simulink model "DC_Charging_Sequence_Block_complete"  (R2025b)
settings: Solver=FixedStepDiscrete  StartTime=0.0  StopTime=10.0  FixedStep=0.01  RelTol=1e-3
undefined symbols (not defined in the file or in its folder): CCM, raptor_get_safe_string, raptor_xcp_function
libraries: Raptor_lib x32
(part 1 of 2)
settings Model: RaptorUIDSize=4  Raptor_Target=CCM-58NN-112-2403  Raptor_Calloc=NonVolatile (EEPROM)  Raptor_ecuaddr=11  RaptorBuildNum=-1  Creator=noahm  LastModifiedBy=nmonson
settings OptimizationCC: DefaultParameterBehavior=Inlined  UseSpecifiedMinMax=on  InlineInvariantSignals=on  EnhancedBackFolding=on  PassReuseOutputArgsAs=Individual arguments  InitFltsAndDblsToZero=on  NoFixptDivByZeroProtection=on  EfficientFloat2IntCast=on  OptimizeBlockOrder=speed  DifferentSizesBufferReuse=on  OptimizationCustomize=off  EfficientTunableParamExpr=on
settings DebuggingCC: UnderspecifiedInitializationDetection=Classic  MergeDetectMultiDrivingBlocksExec=none  InheritedTsInSrcMsg=none  ParameterTunabilityLossMsg=error
settings HardwareCC: TargetIntDivRoundTo=Zero  TargetEndianess=BigEndian  ProdEqTarget=off
settings ModelReferenceCC: PropagateSignalLabelsOutOfModel=off
settings SFSimCC: MATLABDynamicMemAlloc=off
settings RTWCC: SystemTargetFile=raptor.tlc  MakeCommand=raptor_make_rtw  TemplateMakefile=raptor_tmf  Description=Raptor (tm)
settings CodeAppCC: ForceParamTrailComments=on  IgnoreCustomStorageClasses=off  MaxIdLength=100.0  OperatorAnnotations=on  SimulinkDataObjDesc=on  SFDataObjDesc=on  InsertBlockDesc=on
settings STFCustomTargetCC: SystemTargetFile=raptor.tlc  TargetLangStandard=C99 (ISO)  MultiwordLength=256.0  GenerateSampleERTMain=on  ConcurrentExecutionCompliant=off  CombineOutputUpdateFcns=on  CombineSignalStateStructs=on  ERTCustomFileBanners=on  SupportComplex=off  SupportContinuousTime=off  SupportNonInlinedSFcns=off  RemoveResetFunc=on  MATLABClassNameForMDSCustomization=Simulink.SoftwareTarget.ERTCustomization  GRTInterface=off  raptor_autosave=on  raptor_pack_rtw=off
settings ERTTargetCC: ERTCustomFileTemplate=example_file_process.tlc  TargetLangStandard=C99 (ISO)  GenerateSampleERTMain=on  ParMdlRefBuildCompliant=off  CompOptLevelCompliant=off  ConcurrentExecutionCompliant=off  CombineSignalStateStructs=on  SupportComplex=off  ModelStepFunctionPrototypeControlCompliant=off  CPPClassGenCompliant=off  UseToolchainInfoCompliant=off

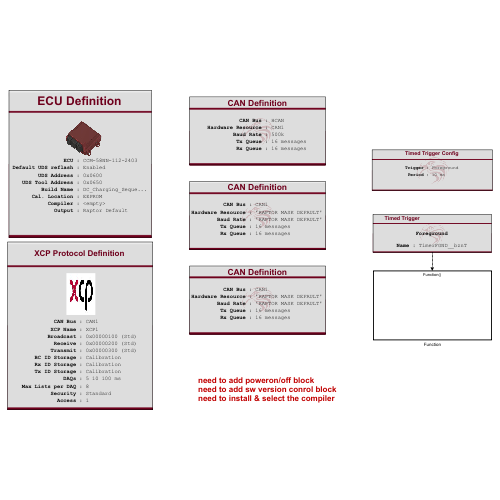
[thumbnail: Simulink's stored preview of the top-level diagram]
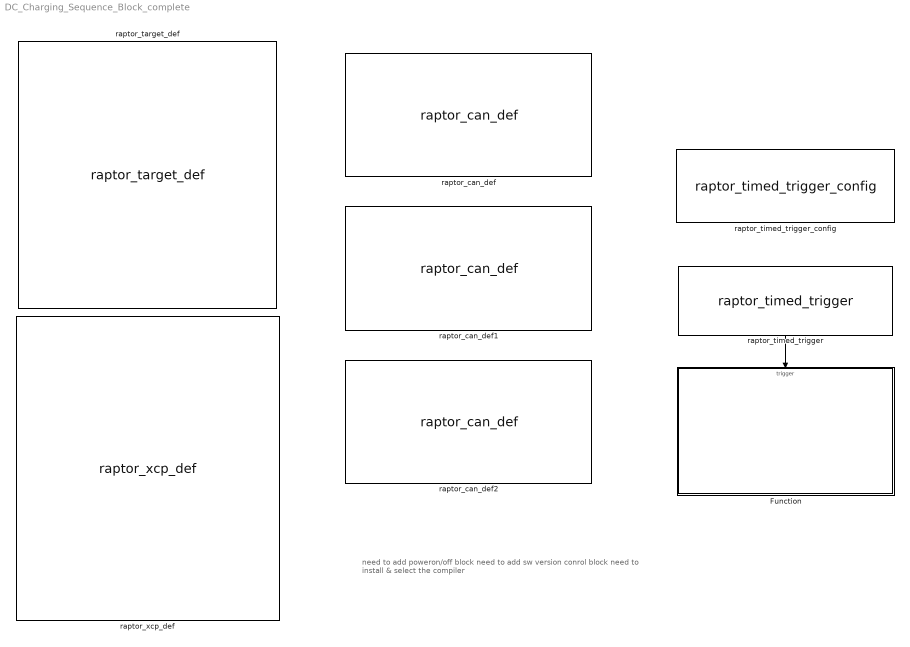
== system DC_Charging_Sequence_Block_complete ==
  note: need to add poweron/off block
      | need to add sw version conrol block
      | need to install & select the compiler
  Function : Subsystem
  raptor_can_def : Raptor_lib/CAN/raptor_can_def  canBus='HCAN'  resourceValues=CAN1|CAN2|CAN3|CAN4|CAN5|CAN6|CAN7|CAN8|(None)  resource=CAN1  baudRateValues=33k|50k|100k|125k|200k|250k|333k|500k|667k|800k|1000k  baudRate=500k  useCustomBR=0  customBR='CustomBaudRate'  enable_baud_rate_config=0  sim_func_name='ConfigureCANBaudRate'  createButton=0  updateButton=0  txQueueSize=16  rxQueueSize=16
      settings: SourceProductName=Raptor
  raptor_can_def1 : Raptor_lib/CAN/raptor_can_def  canBus='CAN1'  resourceValues=CAN1|CAN2|CAN3|CAN4|CAN5|CAN6|CAN7|CAN8|(None)  resource='RAPTOR MASK DEFAULT'  baudRateValues=(None)  baudRate='RAPTOR MASK DEFAULT'  useCustomBR=0  customBR='CustomBaudRate'  enable_baud_rate_config=0  sim_func_name='ConfigureCANBaudRate'  createButton=[]  updateButton=[]  txQueueSize=16  rxQueueSize=16
      settings: SourceProductName=Raptor
  raptor_can_def2 : Raptor_lib/CAN/raptor_can_def  canBus='CAN1'  resourceValues=CAN1|CAN2|CAN3|CAN4|CAN5|CAN6|CAN7|CAN8|(None)  resource='RAPTOR MASK DEFAULT'  baudRateValues=(None)  baudRate='RAPTOR MASK DEFAULT'  useCustomBR=0  customBR='CustomBaudRate'  enable_baud_rate_config=0  sim_func_name='ConfigureCANBaudRate'  createButton=[]  updateButton=[]  txQueueSize=16  rxQueueSize=16
      settings: SourceProductName=Raptor
  raptor_target_def : Raptor_lib/Configuration/raptor_target_def  targetValues=CCM-58NN-112-2403|CCM-TC377-112-2403|DISP-VC128-1901|DISP-VC320L-1402|DISP-VC320-1204|DISP-VC800-1402|DISP-VC500-1904|DISP-VC700-2003|DISP-VC300R-2004|GCM-5634M-070-1559|GCM-5634M-070-1562|EOL-58NN-176-2204|ECM-1793-196-1503|GCM-1793-196-1503|GCM-5605B-048-1906|GCM-5605B-048-2104|RCM-5743R-080-2203|RCM-5743R-080-2304|UAS-5743R-047-2102|UAS-5743R-047-2107|RCM-58NN-112-2103|RCM-58NN-112-2202|RCM-58NN-112-2208|RCM-58NN-112-2410|GCM-TC234-044-2409|GCM-TC277-106-2407|GCM-TC277-108-2406|GCM-TC337-056-2402|GCM-TC367-111-2301|HCM-5604-036-1303|HCM-5604-036-1702  target=CCM-58NN-112-2403  simpack=0  simulator=0  heap=2*1024  stack=4*1024  fgndStack=2*1024  bgndStack=2*1024  idleStack=1024  intStack=1536  sdStack=1024  appStack=1024  ecuaddr=11  disable_def_uds_reflash=0  uds_server_addr_ext=0  uds_server_addr=hex2dec('600')  uds_client_addr=hex2dec('650')  callocValues=Constant (FLASH)|NonVolatile (EEPROM)  calloc=NonVolatile (EEPROM)  compilerValues=[]  compiler=<empty>  setFileName=0  exeName=[raptor_get_safe_string(bdroot) '_']  addBuildNum=0  minVerChars=3  extraOutput=1  buildLocationValues=Raptor Default|Model Directory|User Defined  buildLocation=Raptor Default  exeLocation=''  exeFileButton=0  a2lLocation=''  a2lFileButton=0  rpgLocation=''  rpgFileButton=0
      settings: SourceProductName=Raptor
  raptor_timed_trigger : Raptor_lib/Triggers/raptor_timed_trigger  triggerValues=[]  trigger=Foreground  inherited=0  alwaysEnabled=1  triggerPriority=0  triggerName=FGND__bznT
      settings: SourceProductName=Raptor
  raptor_timed_trigger_config : Raptor_lib/Triggers/raptor_timed_trigger_config  triggerValues=Foreground|Background  trigger=Foreground  period=10
      settings: SourceProductName=Raptor
  raptor_xcp_def : Raptor_lib/Configuration/raptor_xcp_def  XCPname='XCP1'  canBus='CAN1'  bcID=hex2dec('100')  bcID_TypeValues=[]  bcID_Type=Standard  rxID=hex2dec('200')  rxID_TypeValues=[]  rxID_Type=Standard  txID=hex2dec('300')  txID_TypeValues=[]  txID_Type=Standard  daqRates=[5 10 100]  numODTs=8  genCANAPE=0  genVISION=0  securityValues=[]  security=Standard  dllName=raptor_XCPSecurity.dll  accessValues=[]  access=1  bcStorageValues=[]  bcStorage=Calibration  txStorageValues=[]  txStorage=Calibration  rxStorageValues=[]  rxStorage=Calibration
      settings: SourceProductName=Raptor
  wires:
  raptor_timed_trigger/1 -> Function/Trigger

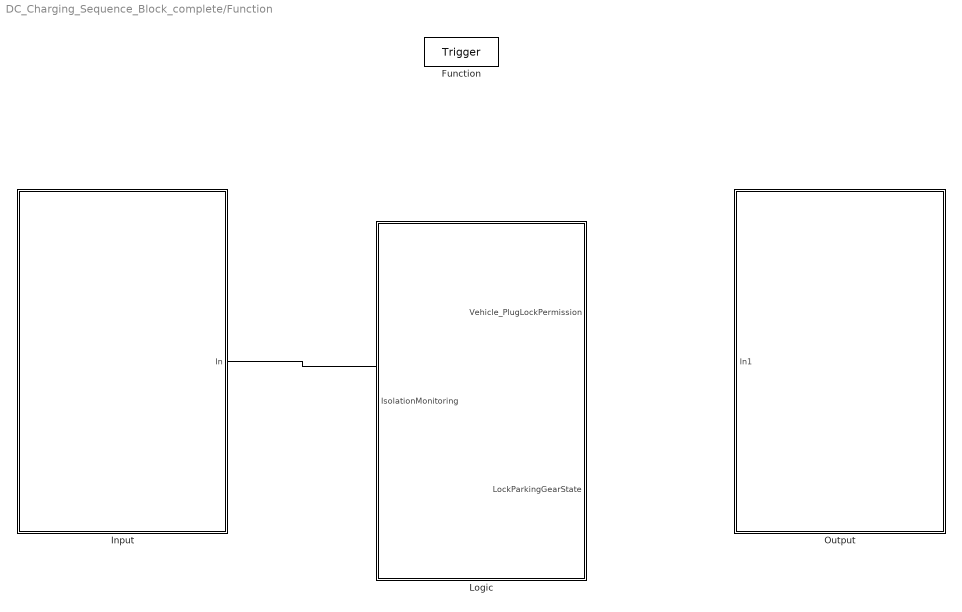
== system DC_Charging_Sequence_Block_complete/Function ==
  Function : TriggerPort  TriggerType=function-call  VariantControl=(inherit)  PortDimensions=1
  Input : Subsystem
  Logic : Subsystem
  Output : Subsystem
  wires:
  Input/1(In) -> ?
  ? -> Output/1(In1)

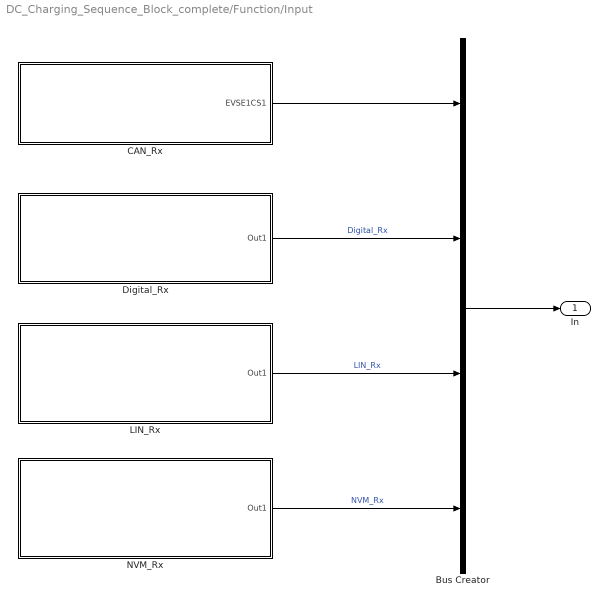
== system DC_Charging_Sequence_Block_complete/Function/Input ==
  Bus Creator : BusCreator  Inputs=4
  CAN_Rx : Subsystem
  Digital_Rx : Subsystem
  LIN_Rx : Subsystem
  NVM_Rx : Subsystem
  In : Outport
  wires:
  Digital_Rx/1(Out1) -> Bus Creator/2  "Digital_Rx"
  LIN_Rx/1(Out1) -> Bus Creator/3  "LIN_Rx"
  NVM_Rx/1(Out1) -> Bus Creator/4  "NVM_Rx"
  Bus Creator/1 -> In/1
  CAN_Rx/1(EVSE1CS1) -> Bus Creator/1

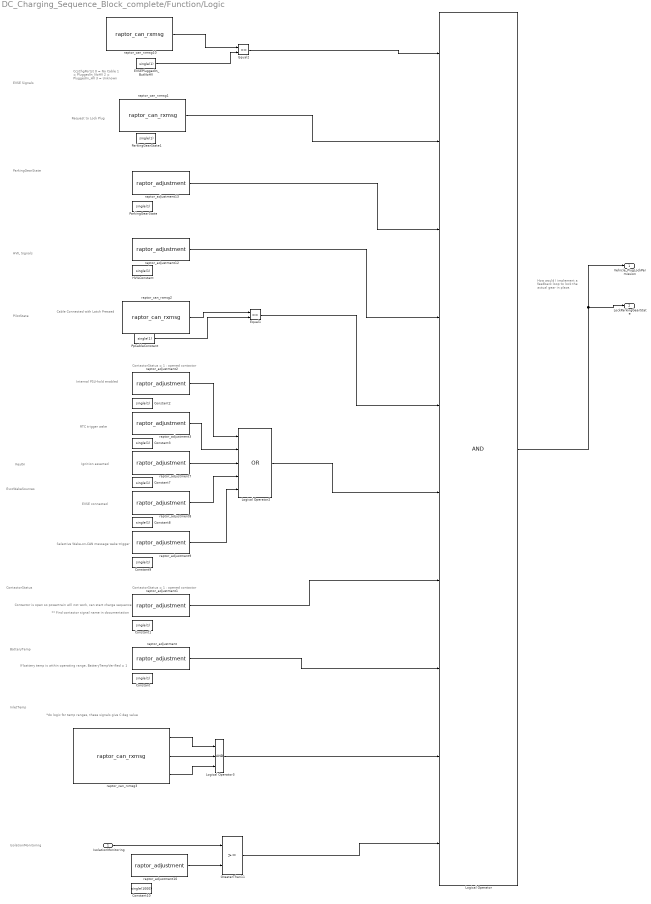
== system DC_Charging_Sequence_Block_complete/Function/Logic ==
  note: Selective Wake-on-CAN message wake trigger
  note: EVSE connected
  note: Ignition asserted
  note: RTC trigger wake
  note: Internal PSU-hold enabled
  note: *do logic for temp ranges, these signals give C deg value
  note: If battery temp is within operating range, BatteryTempVerified = 1
  note: ContactorStatus
  note: EVSE Signals
  note: ParkingGearState
  note: How would I implement a feedback loop to lock the actual gear in place.
  note: Request to Lock Plug
  note: HVIL Signals
  note: PilotState
  note: KeyOn
  note: EvccWakeSources
  note: Contactor is open so powertrain will not work, can start charge sequence
  note: ContactorStatus = 1 : opened contactor
  note: ** Find contactor signal name in documentation
  note: BatteryTemp
  note: InletTemp
  note: IsolationMonitoring
  note: ContactorStatus = 1 : opened contactor
  note: Cable Connected with Latch Pressed
  note: CcsChgPortst
      | 0 = No Cable
      | 1 = PluggedIn_NoHV
      | 2 = PluggedIn_HV
      | 3 = Unknown
  IsolationMonitoring : Inport
  Constant{,1..3,7..9} (7 alike) : Constant  Value=single(1)
  Constant10 : Constant  Value=single(1000)
  EVSEPluggedIn_ButNoHV : Constant  Value=single(1)
  Equal1 : RelationalOperator  Operator===  OutDataTypeStr=boolean  RndMeth=Simplest  InputSameDT=off
  Equal2 : RelationalOperator  Operator===  OutDataTypeStr=boolean  RndMeth=Simplest  InputSameDT=off
  GreaterThan11 : RelationalOperator  OutDataTypeStr=boolean  RndMeth=Simplest  InputSameDT=off
  HVILConstant : Constant  Value=single(1)
  Logical Operator : Logic  Inputs=10  AllPortsSameDT=off  OutDataTypeStr=boolean
  Logical Operator2 : Logic  Operator=OR  Inputs=5  AllPortsSameDT=off  OutDataTypeStr=boolean
  Logical Operator3 : Logic  Inputs=3  AllPortsSameDT=off  OutDataTypeStr=boolean
  ParkingGearState : Constant  Value=single(1)
  ParkingGearState1 : Constant  Value=single(1)
  PpCableConstant : Constant  Value=single(1)
  raptor_adjustment : Raptor_lib/Data Storage/raptor_adjustment  paramName='BatteryTempVerified'  nameSource=Parameter  initValue=1  dataType=single  storage=Calibration  calDispType=Number  calEnum={'False', 'True'}  calGain=1.0  calOffset=0.0  calMax=inf  calMin=-inf  calFormat='-1'  calUnit=''  calHelp=''  calAccess=1  calFunction=raptor_xcp_function(gcb)  calDispHeaders=off  calColHeaders={'Col1' 'Col2' 'Col3'}  calRowHeaders={'Row1' 'Row2' 'Row3'}
      settings: SourceProductName=Raptor
  raptor_adjustment1 : Raptor_lib/Data Storage/raptor_adjustment  paramName='ContactorStatus1'  nameSource=Parameter  initValue=1  dataType=single  storage=Calibration  calDispType=Number  calEnum={'False', 'True'}  calGain=1.0  calOffset=0.0  calMax=inf  calMin=-inf  calFormat='-1'  calUnit=''  calHelp=''  calAccess=1  calFunction=raptor_xcp_function(gcb)  calDispHeaders=off  calColHeaders={'Col1' 'Col2' 'Col3'}  calRowHeaders={'Row1' 'Row2' 'Row3'}
      settings: SourceProductName=Raptor
  raptor_adjustment10 : Raptor_lib/Data Storage/raptor_adjustment  paramName='IsolationMonitoringConstant'  nameSource=Parameter  initValue=1000  dataType=single  storage=Calibration  calDispType=Number  calEnum={'False', 'True'}  calGain=1.0  calOffset=0.0  calMax=inf  calMin=-inf  calFormat='-1'  calUnit=''  calHelp=''  calAccess=1  calFunction=raptor_xcp_function(gcb)  calDispHeaders=off  calColHeaders={'Col1' 'Col2' 'Col3'}  calRowHeaders={'Row1' 'Row2' 'Row3'}
      settings: SourceProductName=Raptor
  raptor_adjustment12 : Raptor_lib/Data Storage/raptor_adjustment  paramName='HVIL_sim'  nameSource=Parameter  initValue=1  dataType=single  storage=Calibration  calDispType=Enumeration  calEnum={'Cable Disconnected', 'Cable Connected with Latch Pressed', 'Cable Connected with Latch Released', 'Proximity Signal is invalid'}  calGain=1.0  calOffset=0.0  calMax=inf  calMin=-inf  calFormat='-1'  calUnit=''  calHelp=''  calAccess=1  calFunction=raptor_xcp_function(gcb)  calDispHeaders=off  calColHeaders={'Col1' 'Col2' 'Col3'}  calRowHeaders={'Row1' 'Row2' 'Row3'}
      settings: SourceProductName=Raptor
  raptor_adjustment13 : Raptor_lib/Data Storage/raptor_adjustment  paramName='ParkingGear_sim'  nameSource=Parameter  initValue=1  dataType=single  storage=Calibration  calDispType=Enumeration  calEnum={'Cable Disconnected', 'Cable Connected with Latch Pressed', 'Cable Connected with Latch Released', 'Proximity Signal is invalid'}  calGain=1.0  calOffset=0.0  calMax=inf  calMin=-inf  calFormat='-1'  calUnit=''  calHelp=''  calAccess=1  calFunction=raptor_xcp_function(gcb)  calDispHeaders=off  calColHeaders={'Col1' 'Col2' 'Col3'}  calRowHeaders={'Row1' 'Row2' 'Row3'}
      settings: SourceProductName=Raptor
  raptor_adjustment2 : Raptor_lib/Data Storage/raptor_adjustment  paramName='EvccWakeSources1_sim'  nameSource=Parameter  initValue=1  dataType=single  storage=Calibration  calDispType=Number  calEnum={'False', 'True'}  calGain=1.0  calOffset=0.0  calMax=inf  calMin=-inf  calFormat='-1'  calUnit=''  calHelp=''  calAccess=1  calFunction=raptor_xcp_function(gcb)  calDispHeaders=off  calColHeaders={'Col1' 'Col2' 'Col3'}  calRowHeaders={'Row1' 'Row2' 'Row3'}
      settings: SourceProductName=Raptor
  raptor_adjustment3 : Raptor_lib/Data Storage/raptor_adjustment  paramName='EvccWakeSources2_sim'  nameSource=Parameter  initValue=1  dataType=single  storage=Calibration  calDispType=Number  calEnum={'False', 'True'}  calGain=1.0  calOffset=0.0  calMax=inf  calMin=-inf  calFormat='-1'  calUnit=''  calHelp=''  calAccess=1  calFunction=raptor_xcp_function(gcb)  calDispHeaders=off  calColHeaders={'Col1' 'Col2' 'Col3'}  calRowHeaders={'Row1' 'Row2' 'Row3'}
      settings: SourceProductName=Raptor
  raptor_adjustment7 : Raptor_lib/Data Storage/raptor_adjustment  paramName='EvccWakeSources3_sim'  nameSource=Parameter  initValue=1  dataType=single  storage=Calibration  calDispType=Number  calEnum={'False', 'True'}  calGain=1.0  calOffset=0.0  calMax=inf  calMin=-inf  calFormat='-1'  calUnit=''  calHelp=''  calAccess=1  calFunction=raptor_xcp_function(gcb)  calDispHeaders=off  calColHeaders={'Col1' 'Col2' 'Col3'}  calRowHeaders={'Row1' 'Row2' 'Row3'}
      settings: SourceProductName=Raptor
  raptor_adjustment8 : Raptor_lib/Data Storage/raptor_adjustment  paramName='EvccWakeSources4_sim'  nameSource=Parameter  initValue=1  dataType=single  storage=Calibration  calDispType=Number  calEnum={'False', 'True'}  calGain=1.0  calOffset=0.0  calMax=inf  calMin=-inf  calFormat='-1'  calUnit=''  calHelp=''  calAccess=1  calFunction=raptor_xcp_function(gcb)  calDispHeaders=off  calColHeaders={'Col1' 'Col2' 'Col3'}  calRowHeaders={'Row1' 'Row2' 'Row3'}
      settings: SourceProductName=Raptor
  raptor_adjustment9 : Raptor_lib/Data Storage/raptor_adjustment  paramName='EvccWakeSources5_sim'  nameSource=Parameter  initValue=1  dataType=single  storage=Calibration  calDispType=Number  calEnum={'False', 'True'}  calGain=1.0  calOffset=0.0  calMax=inf  calMin=-inf  calFormat='-1'  calUnit=''  calHelp=''  calAccess=1  calFunction=raptor_xcp_function(gcb)  calDispHeaders=off  calColHeaders={'Col1' 'Col2' 'Col3'}  calRowHeaders={'Row1' 'Row2' 'Row3'}
      settings: SourceProductName=Raptor
  raptor_can_rxmsg1 : Raptor_lib/CAN/raptor_can_rxmsg  canDefinition=struct('dbcFile', 'CCU_VehicleInterface_R5371_matlab.dbc','message', 'EVCC_Sequence','comment', '','signals', {{'CcsChgPortLockStReq','CcsChgRlyStReq','CcsEvIsolStopReq','CcsRlyWeldCheckEn','Checksum','Counter'}},'enabled', [ 1 0 0 0 0 0;],'scaled', [ 1 1 1 1 1 1;],'canBus', '''CAN1''','messageID', [ 419414367;],'idMask', [ 536870911;],'payloadMask', [],'payloadValue', [],'period', [ 0;],'mailbox', '''''','queueSize', [ 1;],'label', [ 1;],'ver', [ 2;],'showID', [ 0;],'showRaw', [ 0;],'showRawMsg', [ 0;],'useStartVals', [ 0;],'extendedId', [ 1;],'showAge', [ 0;],'useSimFunc', [ 0;],'sim_func_name', '''''','fill', [ 0;],'editID', [ 0;],'signalOrder', [ 1;],'signalAscDes', [ 1;],'msgLength', [ 3;])  canBus='CAN1'  mailbox=''  payloadMask=[]  payloadValue=[]  idMask=hex2dec('1FFFFFFF')  queueSize=1  showID=0  label=1  fill=0  id=419414367  showRaw=0  showAge=0  signalOrder=1  signalInfo={{struct('Name', 'CcsChgPortLockStReq','StartBit', [ 2;],'SignalSize', [ 2;],'ByteOrder', 'LittleEndian','ValueType', 'Integer','Class', 'uint8','Signed', '0','Factor', [ 1;],'Offset', [ 0;],'Min', [ 0;],'Max', [ 3;],'Units', 'bool','Comment', 'Desired status of charge port lock. TRUE value is a request to lock the port and FALSE value is a request to unlock it','Multiplexor', [ 0;],'Multiplexed', [ 0;],'Muxor_Name', '','MultiplexMode_Min', [],'MultiplexMode_Max', [],'StartVal', [ 0;]),struct('Name', 'CcsChgRlyStReq','StartBit', [ 4;],'SignalSize', [ 2;],'ByteOrder', 'LittleEndian','ValueType', 'Integer','Class', 'uint8','Signed', '0','Factor', [ 1;],'Offset', [ 0;],'Min', [ 0;],'Max', [ 3;],'Units', 'bool','Comment', 'Desired relay status request from PI-EVCC; TRUE value is a request to close the relay;','Multiplexor', [ 0;],'Multiplexed', [ 0;],'Muxor_Name', '','MultiplexMode_Min', [],'MultiplexMode_Max', [],'StartVal', [ 0;]),struct('Name', 'CcsEvIsolStopReq','StartBit', [ 0;],'SignalSize', [ 2;],'ByteOrder', 'LittleEndian','ValueType', 'Integer','Class', 'uint8','Signed', '0','Factor', [ 1;],'Offset', [ 0;],'Min', [ 0;],'Max', [ 3;],'Units', 'bool','Comment', 'TRUE value is a Request from PI-EVCC for EV to stop HV Isolation monitoring','Multiplexor', [ 0;],'Multiplexed', [ 0;],'Muxor_Name', '','MultiplexMode_Min', [],'MultiplexMode_Max', [],'StartVal', [ 0;]),struct('Name', 'CcsRlyWeldCheckEn','StartBit', [ 6;],'SignalSize', [ 2;],'ByteOrder', 'LittleEndian','ValueType', 'Integer','Class', 'uint8','Signed', '0','Factor', [ 1;],'Offset', [ 0;],'Min', [ 0;],'Max', [ 3;],'Units', 'bool','Comment', 'Charging session sequence of events: TRUE value is to notify EV that the logic for relay weld-checking can be executed','Multiplexor', [ 0;],'Multiplexed', [ 0;],'Muxor_Name', '','MultiplexMode_Min', [],'MultiplexMode_Max', [],'StartVal', [ 0;]),struct('Name', 'Checksum','StartBit', [ 16;],'SignalSize', [ 8;],'ByteOrder', 'LittleEndian','ValueType', 'Integer','Class', 'uint8','Signed', '0','Factor', [ 1;],'Offset', [ 0;],'Min', [ 0;],'Max', [ 255;],'Units', 'NU','Comment', 'CAN message checksum','Multiplexor', [ 0;],'Multiplexed', [ 0;],'Muxor_Name', '','MultiplexMode_Min', [],'MultiplexMode_Max', [],'StartVal', [ 0;]),struct('Name', 'Counter','StartBit', [ 12;],'SignalSize', [ 4;],'ByteOrder', 'LittleEndian','ValueType', 'Integer','Class', 'uint8','Signed', '0','Factor', [ 1;],'Offset', [ 0;],'Min', [ 0;],'Max', [ 0;],'Units', '','Comment', 'CAN message sequence counter','Multiplexor', [ 0;],'Multiplexed', [ 0;],'Muxor_Name', '','MultiplexMode_Min', [],'MultiplexMode_Max', [],'StartVal', [ 0;])}}  showRawMsg=0  useSimFunc=0  sim_func_name=''  useStartVals=0  extendedId=1
      settings: SourceProductName=Raptor
  raptor_can_rxmsg10 : Raptor_lib/CAN/raptor_can_rxmsg  canDefinition=struct('dbcFile', 'CCU_VehicleInterface_R5371_matlab.dbc','message', 'EVCC_Status','comment', '','signals', {{'CcsChargingMode','CcsChgPortSt','CcsChgSessionPhase','CcsCpState','CcsSelectedControlMode','CcsSelectedProtocol','CcsSelectedServiceId','Checksum','Counter','FaultCode','FaultWord'}},'enabled', [ 0 1 0 0 0 0 0 0 0 0 0;],'scaled', [ 1 1 1 1 1 1 1 1 1 1 1;],'canBus', '''CAN1''','messageID', [ 419414111;],'idMask', [ 536870911;],'payloadMask', [],'payloadValue', [],'period', [ 0;],'mailbox', '''''','queueSize', [ 1;],'label', [ 1;],'ver', [ 2;],'showID', [ 0;],'showRaw', [ 0;],'showRawMsg', [ 0;],'useStartVals', [ 0;],'extendedId', [ 1;],'showAge', [ 0;],'useSimFunc', [ 0;],'sim_func_name', '''''','fill', [ 0;],'editID', [ 0;],'signalOrder', [ 1;],'signalAscDes', [ 1;],'msgLength', [ 8;])  canBus='CAN1'  mailbox=''  payloadMask=[]  payloadValue=[]  idMask=hex2dec('1FFFFFFF')  queueSize=1  showID=0  label=1  fill=0  id=419414111  showRaw=0  showAge=0  signalOrder=1  signalInfo={{struct('Name', 'CcsChargingMode','StartBit', [ 12;],'SignalSize', [ 4;],'ByteOrder', 'LittleEndian','ValueType', 'Integer','Class', 'uint8','Signed', '0','Factor', [ 1;],'Offset', [ 0;],'Min', [ 0;],'Max', [ 15;],'Units', '','Comment', 'Charging mode identified by EVCC based on Control Pilot (CP) PWM input','Multiplexor', [ 0;],'Multiplexed', [ 0;],'Muxor_Name', '','MultiplexMode_Min', [],'MultiplexMode_Max', [],'StartVal', [ 0;]),struct('Name', 'CcsChgPortSt','StartBit', [ 0;],'SignalSize', [ 2;],'ByteOrder', 'LittleEndian','ValueType', 'Integer','Class', 'uint8','Signed', '0','Factor', [ 1;],'Offset', [ 0;],'Min', [ 0;],'Max', [ 3;],'Units', 'enum','Comment', 'The status of charging port (plugged, unplugged, unknown).','Multiplexor', [ 0;],'Multiplexed', [ 0;],'Muxor_Name', '','MultiplexMode_Min', [],'MultiplexMode_Max', [],'StartVal', [ 0;]),struct('Name', 'CcsChgSessionPhase','StartBit', [ 2;],'SignalSize', [ 6;],'ByteOrder', 'LittleEndian','ValueType', 'Integer','Class', 'uint8','Signed', '0','Factor', [ 1;],'Offset', [ 0;],'Min', [ 0;],'Max', [ 63;],'Units', 'No Unit','Comment', 'a number that indicates the current phase of charging session as well as charging mode (AC or DC). See user guide document to interpret the number','Multiplexor', [ 0;],'Multiplexed', [ 0;],'Muxor_Name', '','MultiplexMode_Min', [],'MultiplexMode_Max', [],'StartVal', [ 0;]),struct('Name', 'CcsCpState','StartBit', [ 8;],'SignalSize', [ 4;],'ByteOrder', 'LittleEndian','ValueType', 'Integer','Class', 'uint8','Signed', '0','Factor', [ 1;],'Offset', [ 0;],'Min', [ 0;],'Max', [ 15;],'Units', '','Comment', 'State of Control Pilot (CP) signal','Multiplexor', [ 0;],'Multiplexed', [ 0;],'Muxor_Name', '','MultiplexMode_Min', [],'MultiplexMode_Max', [],'StartVal', [ 0;]),struct('Name', 'CcsSelectedControlMode','StartBit', [ 51;],'SignalSize', [ 1;],'ByteOrder', 'LittleEndian','ValueType', 'Integer','Class', 'uint8','Signed', '0','Factor', [ 1;],'Offset', [ 0;],'Min', [ 0;],'Max', [ 1;],'Units', '','Comment', 'Control Mode selected during ISO15118-20 HLC session; 1 = Dynamic control mode, 0 = Schedule control mode','Multiplexor', [ 0;],'Multiplexed', [ 0;],'Muxor_Name', '','MultiplexMode_Min', [],'MultiplexMode_Max', [],'StartVal', [ 0;]),struct('Name', 'CcsSelectedProtocol','StartBit', [ 40;],'SignalSize', [ 3;],'ByteOrder', 'LittleEndian','ValueType', 'Integer','Class', 'uint8','Signed', '0','Factor', [ 1;],'Offset', [ 0;],'Min', [ 0;],'Max', [ 7;],'Units', '','Comment', 'Protocol selected after exchanging SupportedAppProtocolReq/Res pair','Multiplexor', [ 0;],'Multiplexed', [ 0;],'Muxor_Name', '','MultiplexMode_Min', [],'MultiplexMode_Max', [],'StartVal', [ 0;]),struct('Name', 'CcsSelectedServiceId','StartBit', [ 43;],'SignalSize', [ 8;],'ByteOrder', 'LittleEndian','ValueType', 'Integer','Class', 'uint8','Signed', '0','Factor', [ 1;],'Offset', [ 0;],'Min', [ 0;],'Max', [ 255;],'Units', '','Comment', 'Service ID selected during an HLC session; DC_Charging (2), DC_BPT (17)','Multiplexor', [ 0;],'Multiplexed', [ 0;],'Muxor_Name', '','MultiplexMode_Min', [],'MultiplexMode_Max', [],'StartVal', [ 0;]),struct('Name', 'Checksum','StartBit', [ 56;],'SignalSize', [ 8;],'ByteOrder', 'LittleEndian','ValueType', 'Integer','Class', 'uint8','Signed', '0','Factor', [ 1;],'Offset', [ 0;],'Min', [ 0;],'Max', [ 255;],'Units', 'NU','Comment', 'CAN message checksum','Multiplexor', [ 0;],'Multiplexed', [ 0;],'Muxor_Name', '','MultiplexMode_Min', [],'MultiplexMode_Max', [],'StartVal', [ 0;]),struct('Name', 'Counter','StartBit', [ 52;],'SignalSize', [ 4;],'ByteOrder', 'LittleEndian','ValueType', 'Integer','Class', 'uint8','Signed', '0','Factor', [ 1;],'Offset', [ 0;],'Min', [ 0;],'Max', [ 0;],'Units', '','Comment', 'CAN message sequence counter','Multiplexor', [ 0;],'Multiplexed', [ 0;],'Muxor_Name', '','MultiplexMode_Min', [],'MultiplexMode_Max', [],'StartVal', [ 0;]),struct('Name', 'FaultCode','StartBit', [ 16;],'SignalSize', [ 16;],'ByteOrder', 'LittleEndian','ValueType', 'Integer','Class', 'uint16','Signed', '0','Factor', [ 1;],'Offset', [ 0;],'Min', [ 0;],'Max', [ 65535;],'Units', 'NU','Comment', 'A code that indicates the presence of an active fault related to communication with EV or PiEVCC pins or any fault that is not directly related to EVSE interface','Multiplexor', [ 0;],'Multiplexed', [ 0;],'Muxor_Name', '','MultiplexMode_Min', [],'MultiplexMode_Max', [],'StartVal', [ 0;]),struct('Name', 'FaultWord','StartBit', [ 32;],'SignalSize', [ 8;],'ByteOrder', 'LittleEndian','ValueType', 'Integer','Class', 'uint8','Signed', '0','Factor', [ 1;],'Offset', [ 0;],'Min', [ 0;],'Max', [ 255;],'Units', 'NU','Comment', 'Fault word with each bit representing a particular type of fault','Multiplexor', [ 0;],'Multiplexed', [ 0;],'Muxor_Name', '','MultiplexMode_Min', [],'MultiplexMode_Max', [],'StartVal', [ 0;])}}  showRawMsg=0  useSimFunc=0  sim_func_name=''  useStartVals=0  extendedId=1
      settings: SourceProductName=Raptor
  raptor_can_rxmsg2 : Raptor_lib/CAN/raptor_can_rxmsg  canDefinition=struct('dbcFile', 'CCU_VehicleInterface_R5371_matlab.dbc','message', 'EVCC_IOandWake_Info','comment', '','signals', {{'CcsPpState','Checksum','Counter','Din2St','DoutHsd1St','DoutHsd2St','DoutLsd1St','DoutLsd2St','DoutLsd3St','DoutLsd4St','DoutLsd5St','EvccWakeSources','Hbrg1_Curr','InletLockSt','Rly1FdbkSt','Rly2FdbkSt'}},'enabled', [ 1 0 0 0 0 0 0 0 0 0 0 0 0 0 0 0;],'scaled', [ 1 1 1 1 1 1 1 1 1 1 1 1 1 1 1 1;],'canBus', '''CAN1''','messageID', [ 419416671;],'idMask', [ 536870911;],'payloadMask', [],'payloadValue', [],'period', [ 0;],'mailbox', '''''','queueSize', [ 1;],'label', [ 1;],'ver', [ 2;],'showID', [ 0;],'showRaw', [ 0;],'showRawMsg', [ 0;],'useStartVals', [ 0;],'extendedId', [ 1;],'showAge', [ 0;],'useSimFunc', [ 0;],'sim_func_name', '''''','fill', [ 0;],'editID', [ 0;],'signalOrder', [ 1;],'signalAscDes', [ 1;],'msgLength', [ 7;])  canBus='CAN1'  mailbox=''  payloadMask=[]  payloadValue=[]  idMask=hex2dec('1FFFFFFF')  queueSize=1  showID=0  label=1  fill=0  id=419416671  showRaw=0  showAge=0  signalOrder=1  signalInfo={{struct('Name', 'CcsPpState','StartBit', [ 39;],'SignalSize', [ 3;],'ByteOrder', 'LittleEndian','ValueType', 'Integer','Class', 'uint8','Signed', '0','Factor', [ 1;],'Offset', [ 0;],'Min', [ 0;],'Max', [ 7;],'Units', '','Comment', 'State of Proximity (PP) signal','Multiplexor', [ 0;],'Multiplexed', [ 0;],'Muxor_Name', '','MultiplexMode_Min', [],'MultiplexMode_Max', [],'StartVal', [ 0;]),struct('Name', 'Checksum','StartBit', [ 48;],'SignalSize', [ 8;],'ByteOrder', 'LittleEndian','ValueType', 'Integer','Class', 'uint8','Signed', '0','Factor', [ 1;],'Offset', [ 0;],'Min', [ 0;],'Max', [ 255;],'Units', 'NU','Comment', 'CAN message checksum','Multiplexor', [ 0;],'Multiplexed', [ 0;],'Muxor_Name', '','MultiplexMode_Min', [],'MultiplexMode_Max', [],'StartVal', [ 0;]),struct('Name', 'Counter','StartBit', [ 44;],'SignalSize', [ 4;],'ByteOrder', 'LittleEndian','ValueType', 'Integer','Class', 'uint8','Signed', '0','Factor', [ 1;],'Offset', [ 0;],'Min', [ 0;],'Max', [ 0;],'Units', '','Comment', 'CAN message sequence counter','Multiplexor', [ 0;],'Multiplexed', [ 0;],'Muxor_Name', '','MultiplexMode_Min', [],'MultiplexMode_Max', [],'StartVal', [ 0;]),struct('Name', 'Din2St','StartBit', [ 30;],'SignalSize', [ 2;],'ByteOrder', 'LittleEndian','ValueType', 'Integer','Class', 'uint8','Signed', '0','Factor', [ 1;],'Offset', [ 0;],'Min', [ 0;],'Max', [ 3;],'Units', 'NU','Comment', 'The present state of digital input 2','Multiplexor', [ 0;],'Multiplexed', [ 0;],'Muxor_Name', '','MultiplexMode_Min', [],'MultiplexMode_Max', [],'StartVal', [ 0;]),struct('Name', 'DoutHsd1St','StartBit', [ 26;],'SignalSize', [ 2;],'ByteOrder', 'LittleEndian','ValueType', 'Integer','Class', 'uint8','Signed', '0','Factor', [ 1;],'Offset', [ 0;],'Min', [ 0;],'Max', [ 3;],'Units', 'NU','Comment', 'The present state of HSD digital output 1','Multiplexor', [ 0;],'Multiplexed', [ 0;],'Muxor_Name', '','MultiplexMode_Min', [],'MultiplexMode_Max', [],'StartVal', [ 0;]),struct('Name', 'DoutHsd2St','StartBit', [ 28;],'SignalSize', [ 2;],'ByteOrder', 'LittleEndian','ValueType', 'Integer','Class', 'uint8','Signed', '0','Factor', [ 1;],'Offset', [ 0;],'Min', [ 0;],'Max', [ 3;],'Units', 'NU','Comment', 'The present state of HSD digital output 2','Multiplexor', [ 0;],'Multiplexed', [ 0;],'Muxor_Name', '','MultiplexMode_Min', [],'MultiplexMode_Max', [],'StartVal', [ 0;]),struct('Name', 'DoutLsd1St','StartBit', [ 16;],'SignalSize', [ 2;],'ByteOrder', 'LittleEndian','ValueType', 'Integer','Class', 'uint8','Signed', '0','Factor', [ 1;],'Offset', [ 0;],'Min', [ 0;],'Max', [ 3;],'Units', 'NU','Comment', 'The present state of LSD digital output 1','Multiplexor', [ 0;],'Multiplexed', [ 0;],'Muxor_Name', '','MultiplexMode_Min', [],'MultiplexMode_Max', [],'StartVal', [ 0;]),struct('Name', 'DoutLsd2St','StartBit', [ 18;],'SignalSize', [ 2;],'ByteOrder', 'LittleEndian','ValueType', 'Integer','Class', 'uint8','Signed', '0','Factor', [ 1;],'Offset', [ 0;],'Min', [ 0;],'Max', [ 3;],'Units', 'NU','Comment', 'The present state of LSD digital output 2','Multiplexor', [ 0;],'Multiplexed', [ 0;],'Muxor_Name', '','MultiplexMode_Min', [],'MultiplexMode_Max', [],'StartVal', [ 0;]),struct('Name', 'DoutLsd3St','StartBit', [ 20;],'SignalSize', [ 2;],'ByteOrder', 'LittleEndian','ValueType', 'Integer','Class', 'uint8','Signed', '0','Factor', [ 1;],'Offset', [ 0;],'Min', [ 0;],'Max', [ 3;],'Units', 'NU','Comment', 'The present state of LSD digital output 3','Multiplexor', [ 0;],'Multiplexed', [ 0;],'Muxor_Name', '','MultiplexMode_Min', [],'MultiplexMode_Max', [],'StartVal', [ 0;]),struct('Name', 'DoutLsd4St','StartBit', [ 22;],'SignalSize', [ 2;],'ByteOrder', 'LittleEndian','ValueType', 'Integer','Class', 'uint8','Signed', '0','Factor', [ 1;],'Offset', [ 0;],'Min', [ 0;],'Max', [ 3;],'Units', 'NU','Comment', 'The present state of LSD digital output 4','Multiplexor', [ 0;],'Multiplexed', [ 0;],'Muxor_Name', '','MultiplexMode_Min', [],'MultiplexMode_Max', [],'StartVal', [ 0;]),struct('Name', 'DoutLsd5St','StartBit', [ 24;],'SignalSize', [ 2;],'ByteOrder', 'LittleEndian','ValueType', 'Integer','Class', 'uint8','Signed', '0','Factor', [ 1;],'Offset', [ 0;],'Min', [ 0;],'Max', [ 3;],'Units', 'NU','Comment', 'The present state of LSD digital output 5','Multiplexor', [ 0;],'Multiplexed', [ 0;],'Muxor_Name', '','MultiplexMode_Min', [],'MultiplexMode_Max', [],'StartVal', [ 0;]),struct('Name', 'EvccWakeSources','StartBit', [ 8;],'SignalSize', [ 8;],'ByteOrder', 'LittleEndian','ValueType', 'Integer','Class', 'uint8','Signed', '0','Factor', [ 1;],'Offset', [ 0;],'Min', [ 0;],'Max', [ 255;],'Units', '','Comment', 'Wake sources currently detected by EVCC (bit position based, multiple active possible)','Multiplexor', [ 0;],'Multiplexed', [ 0;],'Muxor_Name', '','MultiplexMode_Min', [],'MultiplexMode_Max', [],'StartVal', [ 0;]),struct('Name', 'Hbrg1_Curr','StartBit', [ 0;],'SignalSize', [ 8;],'ByteOrder', 'LittleEndian','ValueType', 'Integer','Class', 'uint8','Signed', '0','Factor', [ 0.1;],'Offset', [ 0;],'Min', [ 0;],'Max', [ 21;],'Units', 'A','Comment', 'estimated current of H-Bridge 1','Multiplexor', [ 0;],'Multiplexed', [ 0;],'Muxor_Name', '','MultiplexMode_Min', [],'MultiplexMode_Max', [],'StartVal', [ 0;]),struct('Name', 'InletLockSt','StartBit', [ 36;],'SignalSize', [ 3;],'ByteOrder', 'LittleEndian','ValueType', 'Integer','Class', 'uint8','Signed', '0','Factor', [ 1;],'Offset', [ 0;],'Min', [ 0;],'Max', [ 7;],'Units', '','Comment', 'State of the inlet lock','Multiplexor', [ 0;],'Multiplexed', [ 0;],'Muxor_Name', '','MultiplexMode_Min', [],'MultiplexMode_Max', [],'StartVal', [ 0;]),struct('Name', 'Rly1FdbkSt','StartBit', [ 32;],'SignalSize', [ 2;],'ByteOrder', 'LittleEndian','ValueType', 'Integer','Class', 'uint8','Signed', '0','Factor', [ 1;],'Offset', [ 0;],'Min', [ 0;],'Max', [ 3;],'Units', 'NU','Comment', 'Present state of feedback from charge relay/ contactor 1','Multiplexor', [ 0;],'Multiplexed', [ 0;],'Muxor_Name', '','MultiplexMode_Min', [],'MultiplexMode_Max', [],'StartVal', [ 0;]),struct('Name', 'Rly2FdbkSt','StartBit', [ 34;],'SignalSize', [ 2;],'ByteOrder', 'LittleEndian','ValueType', 'Integer','Class', 'uint8','Signed', '0','Factor', [ 1;],'Offset', [ 0;],'Min', [ 0;],'Max', [ 3;],'Units', 'NU','Comment', 'Present state of feedback from charge relay/ contactor 2','Multiplexor', [ 0;],'Multiplexed', [ 0;],'Muxor_Name', '','MultiplexMode_Min', [],'MultiplexMode_Max', [],'StartVal', [ 0;])}}  showRawMsg=0  useSimFunc=0  sim_func_name=''  useStartVals=0  extendedId=1
      settings: SourceProductName=Raptor
  raptor_can_rxmsg3 : Raptor_lib/CAN/raptor_can_rxmsg  canDefinition=struct('dbcFile', 'CCU_VehicleInterface_R5371_matlab.dbc','message', 'EVCC_TempSensor','comment', '','signals', {{'AIN1_Temperature','AIN2_Temperature','AIN3_Temperature','Checksum','Counter'}},'enabled', [ 1 1 1 0 0;],'scaled', [ 1 1 1 1 1;],'canBus', '''CAN1''','messageID', [ 419415903;],'idMask', [ 536870911;],'payloadMask', [],'payloadValue', [],'period', [ 0;],'mailbox', '''''','queueSize', [ 1;],'label', [ 1;],'ver', [ 2;],'showID', [ 0;],'showRaw', [ 0;],'showRawMsg', [ 0;],'useStartVals', [ 0;],'extendedId', [ 1;],'showAge', [ 0;],'useSimFunc', [ 0;],'sim_func_name', '''''','fill', [ 0;],'editID', [ 0;],'signalOrder', [ 1;],'signalAscDes', [ 1;],'msgLength', [ 8;])  canBus='CAN1'  mailbox=''  payloadMask=[]  payloadValue=[]  idMask=hex2dec('1FFFFFFF')  queueSize=1  showID=0  label=1  fill=0  id=419415903  showRaw=0  showAge=0  signalOrder=1  signalInfo={{struct('Name', 'AIN1_Temperature','StartBit', [ 0;],'SignalSize', [ 12;],'ByteOrder', 'LittleEndian','ValueType', 'Integer','Class', 'uint16','Signed', '0','Factor', [ 1;],'Offset', [ -40;],'Min', [ -40;],'Max', [ 4000;],'Units', 'degC_or_Ohm','Comment', 'Temperature measured using AIN1; Typically AC pin temperature at charge inlet; Value can be in Ohm (PTC) or degC (other types such as PT1000, NTC, etc.)','Multiplexor', [ 0;],'Multiplexed', [ 0;],'Muxor_Name', '','MultiplexMode_Min', [],'MultiplexMode_Max', [],'StartVal', [ 40;]),struct('Name', 'AIN2_Temperature','StartBit', [ 12;],'SignalSize', [ 8;],'ByteOrder', 'LittleEndian','ValueType', 'Integer','Class', 'uint8','Signed', '0','Factor', [ 1;],'Offset', [ -40;],'Min', [ -40;],'Max', [ 210;],'Units', 'degC','Comment', 'Temperature measured using AIN 2; Typically DC positive pin temperature at charge inlet','Multiplexor', [ 0;],'Multiplexed', [ 0;],'Muxor_Name', '','MultiplexMode_Min', [],'MultiplexMode_Max', [],'StartVal', [ 40;]),struct('Name', 'AIN3_Temperature','StartBit', [ 20;],'SignalSize', [ 8;],'ByteOrder', 'LittleEndian','ValueType', 'Integer','Class', 'uint8','Signed', '0','Factor', [ 1;],'Offset', [ -40;],'Min', [ -40;],'Max', [ 210;],'Units', 'degC','Comment', 'Temperature measured using AIN3; Typically DC negative pin temperature at charge inlet','Multiplexor', [ 0;],'Multiplexed', [ 0;],'Muxor_Name', '','MultiplexMode_Min', [],'MultiplexMode_Max', [],'StartVal', [ 40;]),struct('Name', 'Checksum','StartBit', [ 56;],'SignalSize', [ 8;],'ByteOrder', 'LittleEndian','ValueType', 'Integer','Class', 'uint8','Signed', '0','Factor', [ 1;],'Offset', [ 0;],'Min', [ 0;],'Max', [ 255;],'Units', 'NU','Comment', 'CAN message checksum','Multiplexor', [ 0;],'Multiplexed', [ 0;],'Muxor_Name', '','MultiplexMode_Min', [],'MultiplexMode_Max', [],'StartVal', [ 0;]),struct('Name', 'Counter','StartBit', [ 52;],'SignalSize', [ 4;],'ByteOrder', 'LittleEndian','ValueType', 'Integer','Class', 'uint8','Signed', '0','Factor', [ 1;],'Offset', [ 0;],'Min', [ 0;],'Max', [ 0;],'Units', '','Comment', 'CAN message sequence counter','Multiplexor', [ 0;],'Multiplexed', [ 0;],'Muxor_Name', '','MultiplexMode_Min', [],'MultiplexMode_Max', [],'StartVal', [ 0;])}}  showRawMsg=0  useSimFunc=0  sim_func_name=''  useStartVals=0  extendedId=1
      settings: SourceProductName=Raptor
  Vehicle_PlugLockPermission : Outport
  LockParkingGearState : Outport  Port=2
  wires:
  Logical Operator/1 -> Vehicle_PlugLockPermission/1, LockParkingGearState/1
  Equal2/1 -> Logical Operator/1
  Logical Operator2/1 -> Logical Operator/6
  raptor_adjustment10/1 -> GreaterThan11/2
  IsolationMonitoring/1 -> GreaterThan11/1
  GreaterThan11/1 -> Logical Operator/10
  raptor_adjustment1/1 -> Logical Operator/7
  raptor_can_rxmsg3/2 -> Logical Operator3/2
  raptor_can_rxmsg3/1 -> Logical Operator3/1
  raptor_can_rxmsg3/3 -> Logical Operator3/3
  raptor_adjustment/1 -> Logical Operator/8
  Logical Operator3/1 -> Logical Operator/9
  raptor_adjustment2/1 -> Logical Operator2/1
  raptor_adjustment3/1 -> Logical Operator2/2
  raptor_adjustment7/1 -> Logical Operator2/3
  raptor_adjustment8/1 -> Logical Operator2/4
  raptor_adjustment9/1 -> Logical Operator2/5
  raptor_can_rxmsg2/1 -> Equal1/1
  PpCableConstant/1 -> Equal1/2
  Equal1/1 -> Logical Operator/5
  raptor_adjustment12/1 -> Logical Operator/4
  raptor_adjustment13/1 -> Logical Operator/3
  raptor_can_rxmsg1/1 -> Logical Operator/2
  raptor_can_rxmsg10/1 -> Equal2/1
  EVSEPluggedIn_ButNoHV/1 -> Equal2/2

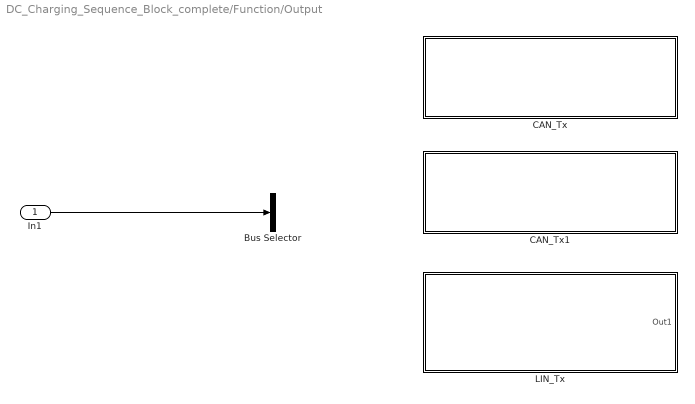
== system DC_Charging_Sequence_Block_complete/Function/Output ==
  In1 : Inport
  Bus Selector : BusSelector  OutputSignals=signal1,signal2
  CAN_Tx : Subsystem
  CAN_Tx1 : Subsystem
  LIN_Tx : Subsystem
  wires:
  In1/1 -> Bus Selector/1

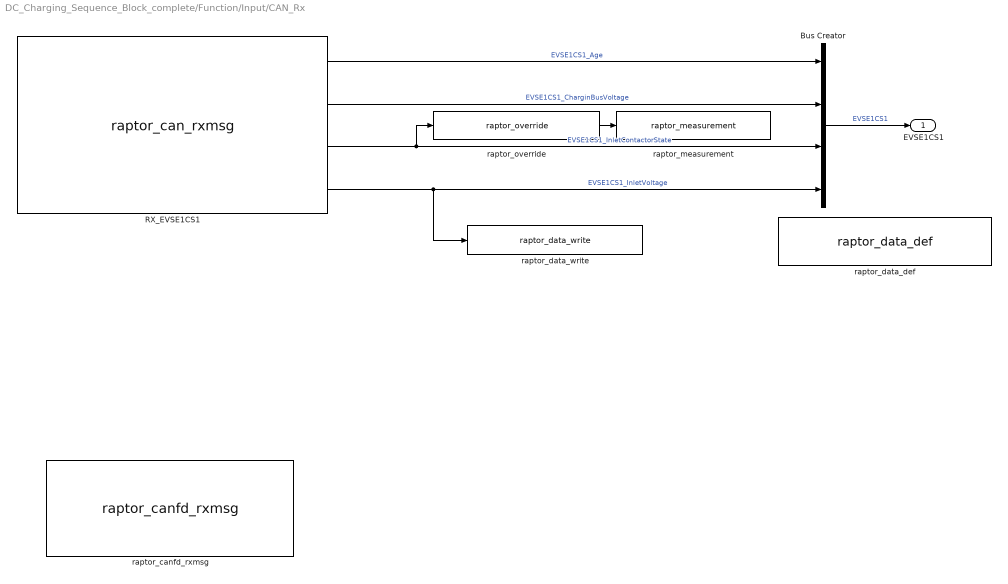
== system DC_Charging_Sequence_Block_complete/Function/Input/CAN_Rx ==
  Bus Creator : BusCreator  Inputs=4
  RX_EVSE1CS1 : Raptor_lib/CAN/raptor_can_rxmsg  canDefinition=struct('dbcFile', 'CCU_VehicleInterface_R5371.dbc','message', 'EVSE1CS1','comment', '','signals', {{'ChargingBusVoltage','InletContactorState','InletVoltage'}},'enabled', [ 1 1 1;],'scaled', [ 1 1 1;],'canBus', '''CAN1''','messageID', [ 419084891;],'idMask', [ 536870911;],'payloadMask', [],'payloadValue', [],'period', [ 0;],'mailbox', '''''','queueSize', [ 1;],'label', [ 0;],'ver', [ 2;],'showID', [ 0;],'showRaw', [ 0;],'showRawMsg', [ 0;],'useStartVals', [ 0;],'extendedId', [ 1;],'showAge', [ 1;],'useSimFunc', [ 0;],'sim_func_name', '''''','fill', [ 0;],'editID', [ 0;],'signalOrder', [ 1;],'signalAscDes', [ 1;],'msgLength', [ 8;])  canBus='CAN1'  mailbox=''  payloadMask=[]  payloadValue=[]  idMask=hex2dec('1FFFFFFF')  queueSize=1  showID=0  label=0  fill=0  id=419084891  showRaw=0  showAge=1  signalOrder=1  signalInfo={{struct('Name', 'InletContactorState','StartBit', [ 32;],'SignalSize', [ 2;],'ByteOrder', 'LittleEndian','ValueType', 'UNSIGNED','Class', 'uint8','Signed', [ 0;],'Factor', [ 1;],'Offset', [ 0;],'Min', [ 0;],'Max', [ 3;],'Units', 'enum','StartVal', [ 0;],'Comment', 'dbc[SPN_13181]','Multiplexed', [ 0;],'Multiplexor', [ 0;],'MultiplexMode_Min', [],'MultiplexMode_Max', []),struct('Name', 'ChargingBusVoltage','StartBit', [ 16;],'SignalSize', [ 16;],'ByteOrder', 'LittleEndian','ValueType', 'UNSIGNED','Class', 'uint16','Signed', [ 0;],'Factor', [ 0.05;],'Offset', [ 0;],'Min', [ 0;],'Max', [ 3276.75;],'Units', 'V','StartVal', [ 0;],'Comment', 'notused[SPN_13180]','Multiplexed', [ 0;],'Multiplexor', [ 0;],'MultiplexMode_Min', [],'MultiplexMode_Max', []),struct('Name', 'InletVoltage','StartBit', [ 0;],'SignalSize', [ 16;],'ByteOrder', 'LittleEndian','ValueType', 'UNSIGNED','Class', 'uint16','Signed', [ 0;],'Factor', [ 0.05;],'Offset', [ 0;],'Min', [ 0;],'Max', [ 3276.75;],'Units', 'V','StartVal', [ 0;],'Comment', 'dbc[SPN_13179]','Multiplexed', [ 0;],'Multiplexor', [ 0;],'MultiplexMode_Min', [],'MultiplexMode_Max', [])}}  showRawMsg=0  useSimFunc=0  sim_func_name=''  useStartVals=0  extendedId=1
      settings: SourceProductName=Raptor
  raptor_canfd_rxmsg : Raptor_lib/CAN/raptor_canfd_rxmsg  canDefinition=struct('dbcFile', 'can_example.dbc','message', 'ExampleMsgTxExtended','comment', 'Example message','signals', {{'Enable','EngineSpeed','EngineTemperature'}},'enabled', [ 1 1 1;],'scaled', [ 1 1 1;],'canBus', '''CAN1''','messageID', [ 777;],'idMask', [ 536870911;],'payloadMask', [],'payloadValue', [],'period', [ 0;],'mailbox', '''''','queueSize', [ 1;],'label', [ 0;],'ver', [ 2;],'showID', [ 0;],'showRaw', [ 0;],'showRawMsg', [ 0;],'showAge', [ 1;],'useSimFunc', [ 0;],'sim_func_name', '''''','enableBRS', [ 0;],'fill', [ 0;],'editID', [ 0;],'signalOrder', [ 1;],'signalAscDes', [ 1;],'msgLength', [ 8;])  canBus='CAN1'  mailbox=''  payloadMask=[]  payloadValue=[]  idMask=hex2dec('1FFFFFFF')  queueSize=1  showID=0  label=0  fill=0  id=777  showRaw=0  showAge=1  signalOrder=1  signalInfo={{struct('Name', 'Enable','StartBit', [ 0;],'SignalSize', [ 1;],'ByteOrder', 'BigEndian','ValueType', 'UNSIGNED','Class', 'uint8','Signed', [ 0;],'Factor', [ 1;],'Offset', [ 0;],'Min', [ 0;],'Max', [ 1;],'Units', '','StartVal', [ 0;],'Comment', '','Multiplexed', [ 0;],'Multiplexor', [ 0;],'MultiplexMode_Min', [],'MultiplexMode_Max', []),struct('Name', 'EngineSpeed','StartBit', [ 16;],'SignalSize', [ 16;],'ByteOrder', 'BigEndian','ValueType', 'UNSIGNED','Class', 'uint16','Signed', [ 0;],'Factor', [ 0.1;],'Offset', [ 0;],'Min', [ 0;],'Max', [ 6500;],'Units', 'rpm','StartVal', [ 0;],'Comment', '','Multiplexed', [ 0;],'Multiplexor', [ 0;],'MultiplexMode_Min', [],'MultiplexMode_Max', []),struct('Name', 'EngineTemperature','StartBit', [ 32;],'SignalSize', [ 16;],'ByteOrder', 'BigEndian','ValueType', 'UNSIGNED','Class', 'uint16','Signed', [ 0;],'Factor', [ 0.01;],'Offset', [ -40;],'Min', [ -40;],'Max', [ 500;],'Units', 'degC','StartVal', [ 0;],'Comment', '','Multiplexed', [ 0;],'Multiplexor', [ 0;],'MultiplexMode_Min', [],'MultiplexMode_Max', [])}}  showRawMsg=0  useSimFunc=0  sim_func_name=''  useStartVals=0  showFD=0  fdEnable=0  showBRS=0  brsEnable=0  extendedId=1
      settings: SourceProductName=Raptor
  raptor_data_def : Raptor_lib/Data Storage/raptor_data_def  dataName='EVSE_InletVoltage'  initValue=0  dataType=single  storage=Volatile (RAM)  calVisible=on  calType=Measurement  calDispType=Number  calEnum={'False', 'True'}  calGain=1.0  calOffset=0  calMin=-inf  calMax=inf  calFormat='-1'  calUnit=''  calHelp=''  calAccess=1  calFunction=raptor_xcp_function(gcb)  calDispHeaders=off  calColHeaders={'Col1' 'Col2' 'Col3'}  calRowHeaders={'Row1' 'Row2' 'Row3'}
      settings: SourceProductName=Raptor
  raptor_data_write : Raptor_lib/Data Storage/raptor_data_write  dataName='EVSE_InletVoltage'  dataShape=Scalar  idxSource=Input Port  idxRow=1  idxCol=1
      settings: SourceProductName=Raptor
  raptor_measurement : Raptor_lib/Data Storage/raptor_measurement  paramName='EVSE_Inlet_Contactor_State'  nameSource=Parameter  calDispType=Number  calEnum={'False', 'True'}  calGain=1.0  calOffset=0.0  calMax=inf  calMin=-inf  calFormat='-1'  calUnit=''  calHelp=''  calAccess=1  calFunction=raptor_xcp_function(gcb)  calVisible=on
      settings: SourceProductName=Raptor
  raptor_override : Raptor_lib/Data Storage/raptor_override  paramName='en_EVSE_Inlet_Contactor_State'  nameSource=Parameter  measurement=None  calDispType=Number  calEnum={'False', 'True'}  calGain=1.0  calOffset=0.0  calMax=inf  calMin=-inf  calFormat='-1'  calUnit=''  calHelp=''  calAccess=1  calFunction="[raptor_xcp_function(gcb) '|'  'Override']"
      settings: SourceProductName=Raptor
  EVSE1CS1 : Outport
  wires:
  RX_EVSE1CS1/3 -> raptor_override/1, Bus Creator/3  "EVSE1CS1_InletContactorState"
  raptor_override/1 -> raptor_measurement/1
  Bus Creator/1 -> EVSE1CS1/1  "EVSE1CS1"
  RX_EVSE1CS1/2 -> Bus Creator/2  "EVSE1CS1_CharginBusVoltage"
  RX_EVSE1CS1/4 -> raptor_data_write/1, Bus Creator/4  "EVSE1CS1_InletVoltage"
  RX_EVSE1CS1/1 -> Bus Creator/1  "EVSE1CS1_Age"

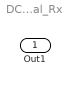
== system DC_Charging_Sequence_Block_complete/Function/Input/Digital_Rx ==
  Out1 : Outport
  wires:
  ? -> Out1/1

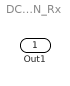
== system DC_Charging_Sequence_Block_complete/Function/Input/LIN_Rx ==
  Out1 : Outport
  wires:
  ? -> Out1/1

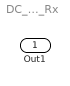
== system DC_Charging_Sequence_Block_complete/Function/Input/NVM_Rx ==
  Out1 : Outport
  wires:
  ? -> Out1/1

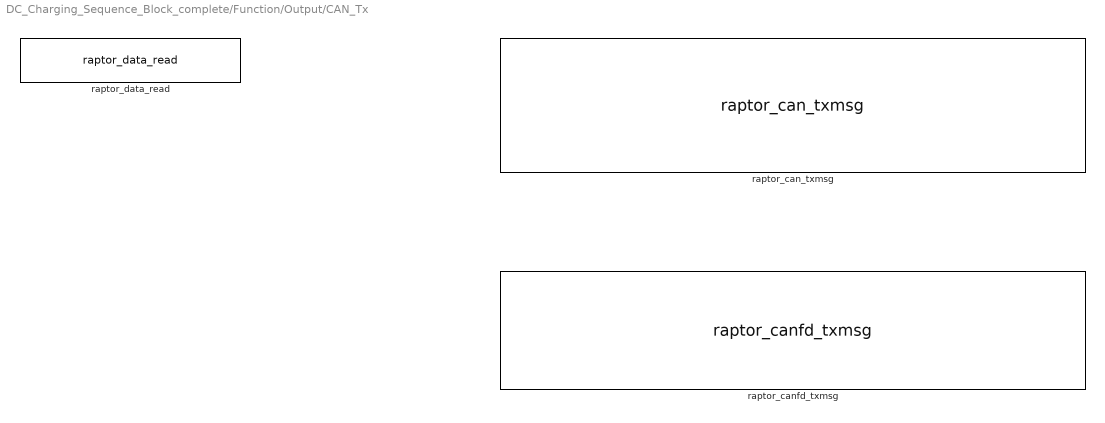
== system DC_Charging_Sequence_Block_complete/Function/Output/CAN_Tx ==
  raptor_can_txmsg : Raptor_lib/CAN/raptor_can_txmsg  canDefinition=struct('dbcFile', '.\CAN\can_example.dbc','message', 'ExampleMsgTxExtended','comment', '','signals', {{'Enable','EngineSpeed','EngineTemperature'}},'enabled', [ 1 1 1;],'canBus', '''CAN1''','messageID', [ 777;],'idMask', [ 536870911;],'payloadMask', [],'payloadValue', [],'period', [ 0;],'mailbox', '','queueSize', [ 1;],'label', [ 0;],'ver', [ 2;],'showID', [ 0;],'showRaw', [ 0;],'fill', [ 0;],'editID', [ 0;],'signalOrder', [ 1;])  canBus='CAN1'  queueSize=1  payloadMask=[]  payloadValue=[]  period=0  showID=0  label=0  idMask=hex2dec('1FFFFFFF')  fill=0  id=777  showRaw=0  signalOrder=1  signalInfo={{struct('Name', 'Enable','StartBit', [ 0;],'SignalSize', [ 1;],'ByteOrder', 'BigEndian','ValueType', 'UNSIGNED','Class', 'uint8','Signed', [ 0;],'Factor', [ 1;],'Offset', [ 0;],'Min', [ 0;],'Max', [ 1;],'Units', '','StartVal', [ 0;],'Comment', '','Multiplexed', [ 0;],'Multiplexor', [ 0;],'MultiplexMode_Min', [],'MultiplexMode_Max', []),struct('Name', 'EngineSpeed','StartBit', [ 16;],'SignalSize', [ 16;],'ByteOrder', 'BigEndian','ValueType', 'UNSIGNED','Class', 'uint16','Signed', [ 0;],'Factor', [ 0.1;],'Offset', [ 0;],'Min', [ 0;],'Max', [ 6500;],'Units', 'rpm','StartVal', [ 0;],'Comment', '','Multiplexed', [ 0;],'Multiplexor', [ 0;],'MultiplexMode_Min', [],'MultiplexMode_Max', []),struct('Name', 'EngineTemperature','StartBit', [ 32;],'SignalSize', [ 16;],'ByteOrder', 'BigEndian','ValueType', 'UNSIGNED','Class', 'uint16','Signed', [ 0;],'Factor', [ 0.01;],'Offset', [ -40;],'Min', [ -40;],'Max', [ 500;],'Units', 'degC','StartVal', [ 0;],'Comment', '','Multiplexed', [ 0;],'Multiplexor', [ 0;],'MultiplexMode_Min', [],'MultiplexMode_Max', [])}}  useSimFunc=0  sim_func_name=''  useStartVals=0
      settings: SourceProductName=Raptor
  raptor_canfd_txmsg : Raptor_lib/CAN/raptor_canfd_txmsg  canDefinition=struct('dbcFile', '.\CAN\can_example.dbc','message', 'ExampleMsgTxExtended','comment', '','signals', {{'Enable','EngineSpeed','EngineTemperature'}},'enabled', [ 1 1 1;],'canBus', '''CAN1''','messageID', [ 777;],'idMask', [ 536870911;],'payloadMask', [],'payloadValue', [],'period', [ 0;],'mailbox', '','queueSize', [ 1;],'label', [ 0;],'ver', [ 2;],'showID', [ 0;],'showRaw', [ 0;],'fill', [ 0;],'editID', [ 0;],'signalOrder', [ 1;])  canBus='CAN1'  queueSize=1  payloadMask=[]  payloadValue=[]  period=0  showID=0  label=0  idMask=hex2dec('1FFFFFFF')  fill=0  id=777  showRaw=0  signalOrder=1  signalInfo={{struct('Name', 'Enable','StartBit', [ 0;],'SignalSize', [ 1;],'ByteOrder', 'BigEndian','ValueType', 'UNSIGNED','Class', 'uint8','Signed', [ 0;],'Factor', [ 1;],'Offset', [ 0;],'Min', [ 0;],'Max', [ 1;],'Units', '','StartVal', [ 0;],'Comment', '','Multiplexed', [ 0;],'Multiplexor', [ 0;],'MultiplexMode_Min', [],'MultiplexMode_Max', []),struct('Name', 'EngineSpeed','StartBit', [ 16;],'SignalSize', [ 16;],'ByteOrder', 'BigEndian','ValueType', 'UNSIGNED','Class', 'uint16','Signed', [ 0;],'Factor', [ 0.1;],'Offset', [ 0;],'Min', [ 0;],'Max', [ 6500;],'Units', 'rpm','StartVal', [ 0;],'Comment', '','Multiplexed', [ 0;],'Multiplexor', [ 0;],'MultiplexMode_Min', [],'MultiplexMode_Max', []),struct('Name', 'EngineTemperature','StartBit', [ 32;],'SignalSize', [ 16;],'ByteOrder', 'BigEndian','ValueType', 'UNSIGNED','Class', 'uint16','Signed', [ 0;],'Factor', [ 0.01;],'Offset', [ -40;],'Min', [ -40;],'Max', [ 500;],'Units', 'degC','StartVal', [ 0;],'Comment', '','Multiplexed', [ 0;],'Multiplexor', [ 0;],'MultiplexMode_Min', [],'MultiplexMode_Max', [])}}  useSimFunc=0  sim_func_name=''  useStartVals=0  brsEnable=0  fdEnable=false
      settings: SourceProductName=Raptor
  raptor_data_read : Raptor_lib/Data Storage/raptor_data_read  dataName='EVSE_InletVoltage'  dataShape=Scalar  idxSource=Input  idxRow=1  idxCol=1
      settings: SourceProductName=Raptor
